simulink model "BlockDiagramSK"  (R2015a)
settings: Solver=ode45  StartTime=0.0  StopTime=10.0  RelTol=1e-3
undefined symbols (not defined in the file): a, f
settings Model: Creator=abeel  LastModifiedBy=abeel

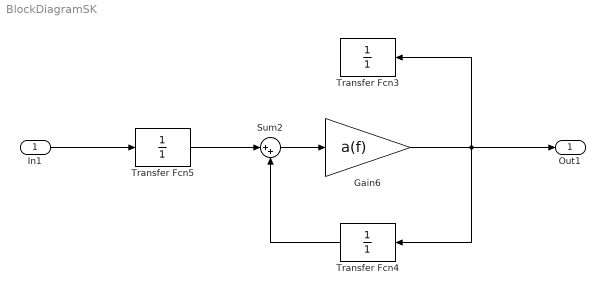
== system BlockDiagramSK ==
  In1 : Inport
  Gain6 : Gain  Gain=a(f)
  Sum2 : Sum  Inputs=|++
  Transfer Fcn3 : TransferFcn  Numerator=1  Denominator=1
  Transfer Fcn4 : TransferFcn  Numerator=1  Denominator=1
  Transfer Fcn5 : TransferFcn  Numerator=1  Denominator=1
  Out1 : Outport
  wires:
  Transfer Fcn5/1 -> Sum2/1
  Sum2/1 -> Gain6/1
  Gain6/1 -> Transfer Fcn3/1, Out1/1, Transfer Fcn4/1
  Transfer Fcn4/1 -> Sum2/2
  In1/1 -> Transfer Fcn5/1
